simulink model "Bldc_hall"  (R2023a)
settings: Solver=VariableStepAuto  StartTime=0.0  StopTime=1  RelTol=1e-3
libraries: spsIGBTDiodeLib x6, spsDCVoltageSourceLib x1, spsPermanentMagnetSynchronousMachineLib x1, spsSeriesRLCBranchLib x1, spspowerguiLib x1
settings Model: Creator=ANKIT  LastModifiedBy=ANKIT

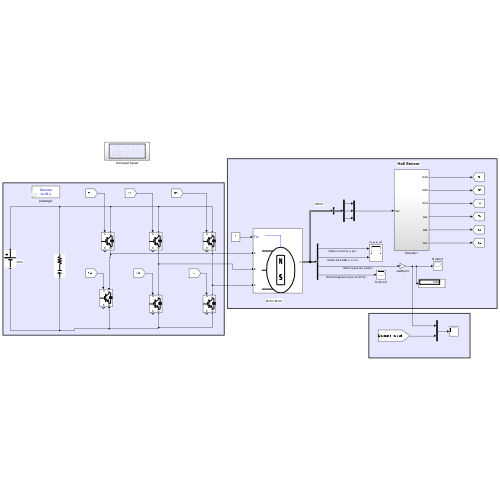
[thumbnail: Simulink's stored preview of the top-level diagram]
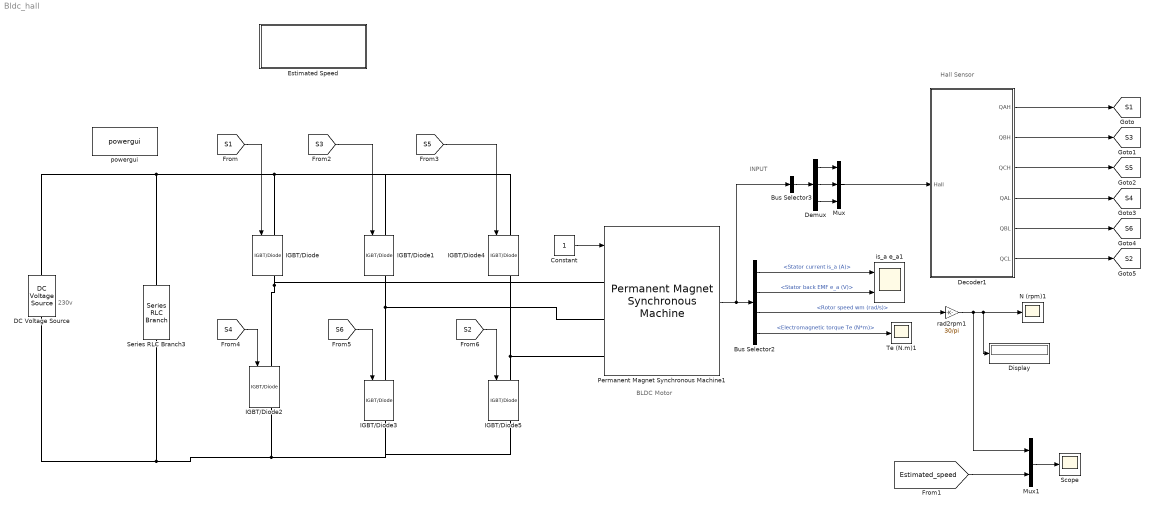
== system Bldc_hall ==
  note: BLDC Motor
  note: 230v
  note: INPUT
  note: Hall Sensor
  Bus Selector2 : BusSelector  OutputSignals=Stator current is_a (A),Stator back EMF e_a (V),Rotor speed wm (rad/s),Electromagnetic torque Te (N*m)
  Bus Selector3 : BusSelector  OutputSignals=Hall effect signal h_a,Hall effect signal h_b,Hall effect signal h_c  OutputAsBus=on
  Constant : Constant
  DC Voltage Source : spsDCVoltageSourceLib/DC Voltage Source  Amplitude=300  Measurements=None
  Decoder1 : Subsystem
  Demux : Demux  Outputs=3
  Display : Display
  Estimated Speed : Subsystem
  IGBT/Diode{,1..5} (6 alike) : spsIGBTDiodeLib/IGBT//Diode  Ron=1e-3  Rs=1e5  Cs=inf  Measurements=on
  Mux : Mux  Inputs=3
  Mux1 : Mux  Inputs=2
  N (rpm)1 : Scope
  Permanent Magnet Synchronous Machine1 : spsPermanentMagnetSynchronousMachineLib/Permanent Magnet Synchronous Machine  NbPhases=3  FluxDistribution=Trapezoidal  RotorType=Round  MechanicalLoad=Torque Tm  PresetModel=No  ShowDetailedParameters=on  MeasurementBus=off  Resistance=2.8750  Inductance=8.5e-3  dqInductances=[8.5e-3, 8.5e-3]  La=0.000835  MachineConstant=Flux linkage established by magnets (V.s)  Flux=0.175  VoltageCst=293.2153  TorqueCst=2.8  Flat=120  Mechanical=[ 0.8e-3, 1e-3 8]  PolePairs=4  InitialConditions=[0,0, 0,0]  InitialConditions5ph=[0 0 0 0 0 0]  RefAngle=90 degrees behind phase A axis (modified Park)  IterativeDiscreteModel=Trapezoidal non iterative  TsBlock=-1  TsPowergui=0
  Scope : Scope
  Series RLC Branch3 : spsSeriesRLCBranchLib/Series RLC Branch  LConnTagsString=__new0  RConnTagsString=__new0  BranchType=RC  Resistance=0.001  Inductance=1e-3  SetiL0=off  InitialCurrent=0  Capacitance=1000e-6  Setx0=off  InitialVoltage=0  Measurements=None
  Te (N.m)1 : Scope
  is_a e_a1 : Scope  NumInputPorts=2
  powergui : spspowerguiLib/powergui  Priority=2  SimulationMode=Discrete  SampleTime=1e-6  frequency=60  Iterations=50  frequencyindice=0  Pbase=100e6  ErrMax=1e-4  UnitsV=kV  UnitsW=MW  buscounter=0  FunctionMessages=off  echomessages=off  EnableUseOfTLC=off  CurrentSourceSwitches=off  DisableSnubberDevices=off  DisableRonSwitches=off  DisableVfSwitches=off  DisplayEquations=off  AutomaticDiscreteSolvers=off  SolverType=Tustin/Backward Euler (TBE)  Interpol=off  ExternalGateDelay=off  methode=off  Ts=0  x0status=blocks  SPID=off  SwTol=0  HookPort=off  NonlinearTolerance=1e-4  nMaxIteration=100  ContinueOnMaxIteration=off  RestoreLinks=warning  ResistiveCurrentMeasurement=off  Frange=[0:2:500]  Ylog=off  Xlog=on  ShowGrid=off  save=off  variable=ZData  structure=0  ZoomFFT=on  StartTime=0.0  cycles=1  DisplayStyle=1  fundamental=60  FreqAxis=off  MaxFrequency=1000  frequencyindicesteady=1  RmsSteady=1  display=off
  rad2rpm1 : Gain  Gain=30/pi
  tag scope: S1=global, S2=global, S3=global, S4=global, S5=global, S6=global
  wires:
  [S1] -> IGBT/Diode/1
  [S6] -> IGBT/Diode3/1
  [S5] -> IGBT/Diode4/1
  [S3] -> IGBT/Diode1/1
  [S2] -> IGBT/Diode5/1
  [S4] -> IGBT/Diode2/1
  Decoder1/2(QBH) -> [S3]
  Decoder1/6(QCL) -> [S2]
  Demux/1 -> Mux/1
  Decoder1/5(QBL) -> [S6]
  Mux/1 -> Decoder1/1("Hall ")
  Demux/2 -> Mux/2
  Decoder1/4(QAL) -> [S4]
  Demux/3 -> Mux/3
  Constant/1 -> Permanent Magnet Synchronous Machine1/1
  Decoder1/1(QAH) -> [S1]
  Permanent Magnet Synchronous Machine1/1 -> Bus Selector3/1, Bus Selector2/1
  Bus Selector2/4 -> Te (N.m)1/1  "<Electromagnetic torque Te (N*m)>"
  Decoder1/3(QCH) -> [S5]
  Bus Selector3/1 -> Demux/1
  Bus Selector2/2 -> is_a e_a1/2  "<Stator back EMF e_a (V)>"
  Bus Selector2/3 -> rad2rpm1/1  "<Rotor speed wm (rad/s)>"
  Bus Selector2/1 -> is_a e_a1/1  "<Stator current is_a (A)>"
  Mux1/1 -> Scope/1
  [Estimated_speed] -> Mux1/2
  rad2rpm1/1 -> Mux1/1, Display/1, N (rpm)1/1
  connections:
  Series RLC Branch3/LConn1 -- IGBT/Diode4/LConn1 -- IGBT/Diode1/LConn1 -- IGBT/Diode/LConn1 -- DC Voltage Source/RConn1
  IGBT/Diode2/RConn1 -- IGBT/Diode3/RConn1 -- IGBT/Diode5/RConn1 -- DC Voltage Source/LConn1 -- Series RLC Branch3/RConn1
  IGBT/Diode/RConn1 -- Permanent Magnet Synchronous Machine1/LConn1 -- IGBT/Diode2/LConn1
  IGBT/Diode3/LConn1 -- Permanent Magnet Synchronous Machine1/LConn2 -- IGBT/Diode1/RConn1
  IGBT/Diode4/RConn1 -- Permanent Magnet Synchronous Machine1/LConn3 -- IGBT/Diode5/LConn1

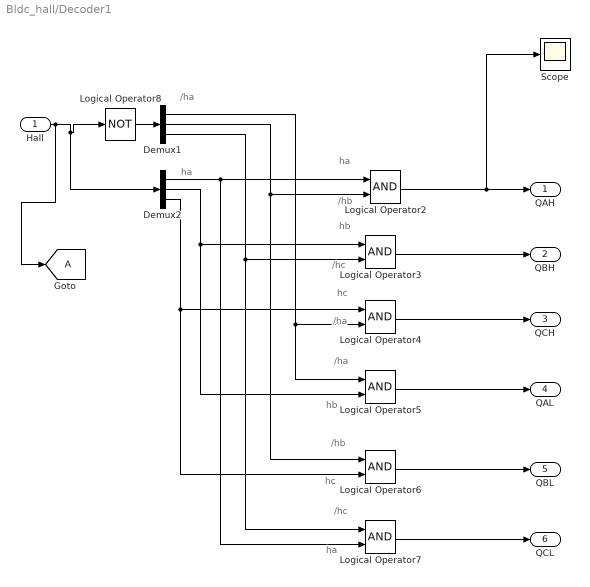
== system Bldc_hall/Decoder1 ==
  note: ha
  note: /hc
  note: hc
  note: /hb
  note: hb
  note: /ha
  note: /ha
  note: hc
  note: /hc
  note: hb
  note: /hb
  note: ha
  note: ha
  note: /ha
  "Hall " : Inport
  Demux1 : Demux  Outputs=3
  Demux2 : Demux  Outputs=3
  Goto : Goto  TagVisibility=global
  Logical Operator{2..7} (6 alike) : Logic  AllPortsSameDT=off  OutDataTypeStr=boolean
  Logical Operator8 : Logic  Operator=NOT  AllPortsSameDT=off  OutDataTypeStr=boolean
  Scope : Scope
  QAH : Outport  VectorParamsAs1DForOutWhenUnconnected=off
  QBH : Outport  Port=2  VectorParamsAs1DForOutWhenUnconnected=off
  QCH : Outport  Port=3  VectorParamsAs1DForOutWhenUnconnected=off
  QAL : Outport  Port=4  VectorParamsAs1DForOutWhenUnconnected=off
  QBL : Outport  Port=5  VectorParamsAs1DForOutWhenUnconnected=off
  QCL : Outport  Port=6  VectorParamsAs1DForOutWhenUnconnected=off
  wires:
  Demux1/1 -> Logical Operator5/1, Logical Operator4/2
  Demux1/2 -> Logical Operator6/1, Logical Operator2/2
  Demux1/3 -> Logical Operator7/1, Logical Operator3/2
  Demux2/1 -> Logical Operator7/2, Logical Operator2/1
  Demux2/2 -> Logical Operator5/2, Logical Operator3/1
  Demux2/3 -> Logical Operator6/2, Logical Operator4/1
  Logical Operator2/1 -> Scope/1, QAH/1
  Logical Operator3/1 -> QBH/1
  Logical Operator4/1 -> QCH/1
  Logical Operator5/1 -> QAL/1
  Logical Operator7/1 -> QCL/1
  "Hall "/1 -> Goto/1, Demux2/1, Logical Operator8/1
  Logical Operator8/1 -> Demux1/1
  Logical Operator6/1 -> QBL/1

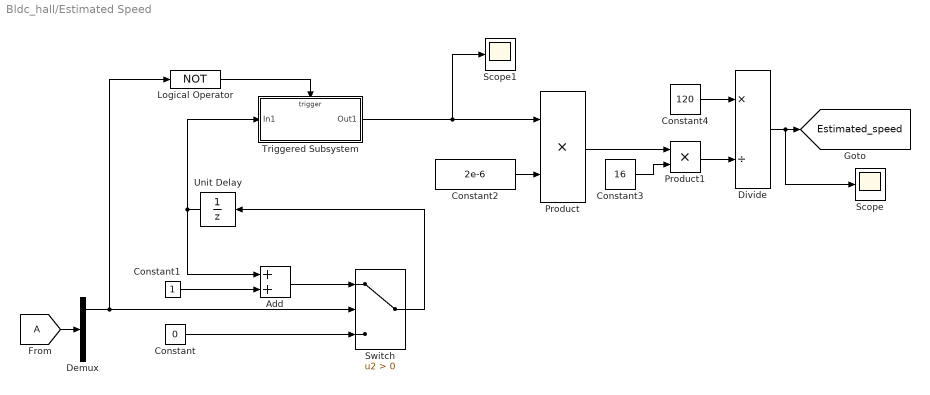
== system Bldc_hall/Estimated Speed ==
  Add : Sum
  Constant : Constant  Value=0
  Constant1 : Constant
  Constant2 : Constant  Value=2e-6
  Constant3 : Constant  Value=16
  Constant4 : Constant  Value=120
  Demux : Demux  Outputs=3
  Divide : Product  Inputs=*/
  From : From  TagVisibility=global
  Logical Operator : Logic  Operator=NOT  AllPortsSameDT=off  OutDataTypeStr=boolean
  Product : Product
  Product1 : Product
  Scope : Scope
  Scope1 : Scope
  Switch : Switch  Criteria=u2 > Threshold  SaturateOnIntegerOverflow=off  InputSameDT=off
  Triggered Subsystem : Subsystem  TreatAsAtomicUnit=on
  Unit Delay : UnitDelay  SampleTime=-1  HasFrameUpgradeWarning=on
  tag scope: Estimated_speed=global
  wires:
  From/1 -> Demux/1
  Constant/1 -> Switch/3
  Switch/1 -> Unit Delay/1
  Demux/1 -> Logical Operator/1, Switch/2
  Unit Delay/1 -> Add/1, Triggered Subsystem/1(In1)
  Constant1/1 -> Add/2
  Add/1 -> Switch/1
  Logical Operator/1 -> Triggered Subsystem/Trigger
  Triggered Subsystem/1(Out1) -> Scope1/1, Product/1
  Constant2/1 -> Product/2
  Product/1 -> Product1/1
  Constant3/1 -> Product1/2
  Product1/1 -> Divide/2
  Constant4/1 -> Divide/1
  Divide/1 -> Scope/1, [Estimated_speed]

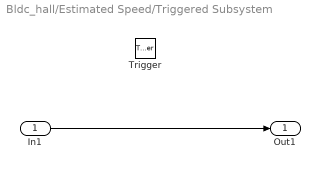
== system Bldc_hall/Estimated Speed/Triggered Subsystem ==
  In1 : Inport
  Trigger : TriggerPort  VariantControl=(inherit)
  Out1 : Outport
  wires:
  In1/1 -> Out1/1
